simulink model "PubIfDecisionTOS_MDL"  (R2020b)
settings: configuration reference "DspaceConfig" (kept outside this file)
PostLoadFcn:
  | if any(exist('dsrtsu_mdlpostloadfcn', 'file') ~= 0), dsrtsu_mdlpostloadfcn('Execute', bdroot); end
InitFcn:
  | , if any(exist('dsmpb_private', 'file') ~= 0), dsmpb_private('dsmpb_mdlclblib', 'Init', bdroot); end,
undefined symbols (not defined in the file or in its folder): C_TOS_ACCEgoRAxletoFbumplength_m, C_TOS_ACCTargetFront_Flag, C_TOS_AEBJAPedObjDxThre_Val, C_TOS_AEBJAPedObjDyThre_Val, C_TOS_AEBJATargetSize_Val, C_TOS_AEBJAVehObjDxThre_Val, C_TOS_AEBJAVehObjDyThre_Val, C_TOS_AEBJuncPedTargetSize_Val, C_TOS_AEBLatObjDxThre_Val, C_TOS_AEBLatPedDyThre_Val, C_TOS_AEBLatTargetSize_Val, C_TOS_AEBLongTargetInEgoFront_Flag, C_TOS_axAbsGround_Parameter, C_TOS_CameraConfirmedFlag, C_TOS_CNsubjWidth, C_TOS_CurrentLaneCoreMinWidth_Val, C_TOS_CutInProb_Val_Zero, C_TOS_CutOutProb_Val_Zero, C_TOS_D2R_Val, C_TOS_DefaultValueObjectToCenterLine_dy, C_TOS_EgoCarWidth_Val, C_TOS_EgoDxRefPoint_m, C_TOS_EgoRAxletoFbumplength_m, C_TOS_HalfWidthVehicle_Con, C_TOS_HWA_CurrentLaneFlag, C_TOS_HWA_LeftLaneFlag, C_TOS_HWA_MovingDir_Vaild, C_TOS_HWA_MovState_Vaild, C_TOS_HWA_RightLaneFlag, C_TOS_LaneLineCourseErrorFront, C_TOS_LaneLineCourseErrorRear, C_TOS_MotorbikeDefaultWidth_m, C_TOS_NumberOfEffectiveTargets, C_TOS_Obj_Age_Val, C_TOS_Objdx_Constraint_Val, C_TOS_ObjectDefaultWidth_m, C_TOS_ObjInCurrentLane_Val, C_TOS_ObjInCurrentLaneValid, C_TOS_ObjInLeftLaneValid, C_TOS_ObjInRightLaneValid, C_TOS_ObjNotInCurrentLane_Val, C_TOS_ObjNotREElementType, C_TOS_ObjPredictDis_dy_ConstantVal_Zeros, C_TOS_ObjToCenterLine_ConstantVal_Zeros, C_TOS_OFMObjIDInvilad_Val, C_TOS_PIL_LatDisCons_Val_zero, C_TOS_PIL_ObjectCutInFlag_b, C_TOS_PIL_ObjectCutOutFlag_b, C_TOS_PIL_ObjLaneProb_al_Val, C_TOS_PP_ObjFusType_FC_Confirm_b, C_TOS_PP_ObjFusType_FC_FR_Confirm_b, C_TOS_PP_ObjFusType_FR_Confirm_b, C_TOS_RE_80BoolDefault_Val, C_TOS_RE_80Single181Default_Val, C_TOS_RE_80Single255Default_Val, C_TOS_RE_80Uint8Default_Val, C_TOS_RE_D2R, C_TOS_RE_D_180_Val, C_TOS_RE_InvalidObjectID_Val, C_TOS_RE_InvalidTargetChainDir_Val ... (+142)
libraries: simulink x1650, TOS_LIB x361, canfdmsglib x14
(part 1 of 69)
PreSaveFcn:
  | , if any(exist('dsmpb_private', 'file') ~= 0), dsmpb_private('dsmpb_mdlclblib', 'PreSave', bdroot); end,
CloseFcn:
  | , if any(exist('dsmpb_private', 'file') ~= 0), dsmpb_private('dsmpb_mdlclblib', 'Close', bdroot); end,
settings Model: DataDictionary=HWA_DDs.sldd  RTICANMMDATA=struct('GeneralSetupData',struct('modelroot','C:\Users\GW00133806\Desktop\ADAS_Store\Project\V61_Autobox_Noa\LM_TOS','generalsettings',struct('filesettings',struct('destfolder',struct('Name','RTICANMM_FILES','Check',1),'buildfolder',struct('Name','.','Check',1),'AbsDestfolder',struct('Name','C:\Users\GW00133806\Desktop\ADAS_Store\Project\V61_Autobox_Noa\LM_TOS\RTICANMM_FILES'),'AbsBuildfolder',struct('Name','C:\Users\GW00133806\Desktop\ADAS_Store\Project\V61_Autobox_Noa\LM_TOS'))),'options',struct('addpaths',1,'rmpaths',1,'addtrcexclusion',false,'cannavigator',struct('checkmonitoring',0),'show_usrtrc',0,'use_usrtrc',0),'advanced',struct('options',ones(1,100)),'MPSetup',{{}},'RTI',struct('Type','DSRT','Ver','4.2','Date','02-Nov-2019'),'modelname','PubIfDecisionTOS_MDL','block','PubIfDecisionTOS_MDL'))  DSRTSU_INTERNAL_RTIFPGA=150  Creator=GW00180895  LastModifiedBy=GW00133806
settings ConfigSetRef: SourceName=DspaceConfig

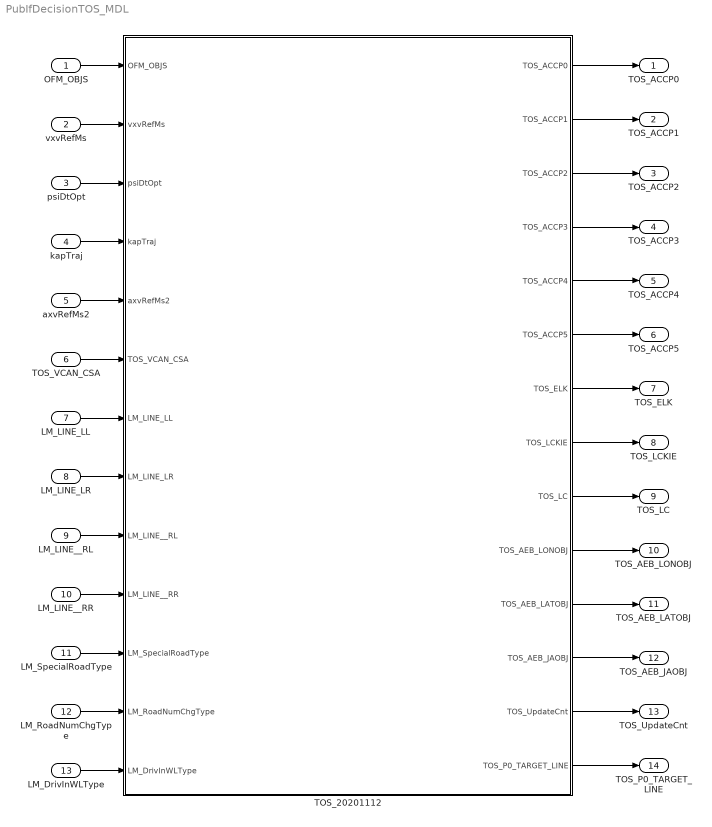
== system PubIfDecisionTOS_MDL ==
  OFM_OBJS : Inport  OutDataTypeStr=Bus: OFM_OBJ_BUS  PortDimensions=1  BusOutputAsStruct=on
  vxvRefMs : Inport  Port=2  OutDataTypeStr=single  PortDimensions=1  BusOutputAsStruct=on
  psiDtOpt : Inport  Port=3  OutDataTypeStr=single  PortDimensions=1  BusOutputAsStruct=on
  kapTraj : Inport  Port=4  OutDataTypeStr=single  PortDimensions=1  BusOutputAsStruct=on
  axvRefMs2 : Inport  Port=5  OutDataTypeStr=single  PortDimensions=1  BusOutputAsStruct=on
  TOS_VCAN_CSA : Inport  Port=6  OutDataTypeStr=Bus: TOS_VCAN_CSA_BUS  BusOutputAsStruct=on
  LM_LINE_LL : Inport  Port=7  OutDataTypeStr=Bus: LM_LINE_BUS  PortDimensions=1  BusOutputAsStruct=on
  LM_LINE_LR : Inport  Port=8  OutDataTypeStr=Bus: LM_LINE_BUS  PortDimensions=1  BusOutputAsStruct=on
  LM_LINE__RL : Inport  Port=9  OutDataTypeStr=Bus: LM_LINE_BUS  PortDimensions=1  BusOutputAsStruct=on
  LM_LINE__RR : Inport  Port=10  OutDataTypeStr=Bus: LM_LINE_BUS  PortDimensions=1  BusOutputAsStruct=on
  LM_SpecialRoadType : Inport  Port=11  OutDataTypeStr=uint8  PortDimensions=1  BusOutputAsStruct=on
  LM_RoadNumChgType : Inport  Port=12  OutDataTypeStr=uint8  PortDimensions=1  BusOutputAsStruct=on
  LM_DrivInWLType : Inport  Port=13  OutDataTypeStr=uint8  PortDimensions=1  BusOutputAsStruct=on
  TOS_20201112 : Subsystem
  TOS_ACCP0 : Outport  OutDataTypeStr=Bus: TOS_ACCP0_BUS  PortDimensions=1  BusOutputAsStruct=on
  TOS_ACCP1 : Outport  Port=2  OutDataTypeStr=Bus: TOS_ACCP1_BUS  PortDimensions=1  BusOutputAsStruct=on
  TOS_ACCP2 : Outport  Port=3  OutDataTypeStr=Bus: TOS_ACCP2_BUS  PortDimensions=1  BusOutputAsStruct=on
  TOS_ACCP3 : Outport  Port=4  OutDataTypeStr=Bus: TOS_ACCP3_BUS  PortDimensions=1  BusOutputAsStruct=on
  TOS_ACCP4 : Outport  Port=5  OutDataTypeStr=Bus: TOS_ACCP4_BUS  PortDimensions=1  BusOutputAsStruct=on
  TOS_ACCP5 : Outport  Port=6  OutDataTypeStr=Bus: TOS_ACCP5_BUS  PortDimensions=1  BusOutputAsStruct=on
  TOS_ELK : Outport  Port=7  OutDataTypeStr=Bus: TOS_ELK_BUS  PortDimensions=1  BusOutputAsStruct=on
  TOS_LCKIE : Outport  Port=8  OutDataTypeStr=Bus: TOS_LCKIE_BUS  PortDimensions=1  BusOutputAsStruct=on
  TOS_LC : Outport  Port=9  OutDataTypeStr=Bus: TOS_LC_BUS  PortDimensions=1  BusOutputAsStruct=on
  TOS_AEB_LONOBJ : Outport  Port=10  OutDataTypeStr=Bus: TOS_AEB_LONOBJ_BUS  PortDimensions=1  BusOutputAsStruct=on
  TOS_AEB_LATOBJ : Outport  Port=11  OutDataTypeStr=Bus: TOS_AEB_LATOBJ_BUS  PortDimensions=10  BusOutputAsStruct=on
  TOS_AEB_JAOBJ : Outport  Port=12  OutDataTypeStr=Bus: TOS_AEB_JAOBJ_BUS  PortDimensions=32  BusOutputAsStruct=on
  TOS_UpdateCnt : Outport  Port=13  OutDataTypeStr=uint32  PortDimensions=1  BusOutputAsStruct=on
  TOS_P0_TARGET_LINE : Outport  Port=14  OutDataTypeStr=Bus: TOS_P0_TARGET_LINE_BUS  PortDimensions=1  BusOutputAsStruct=on
  wires:
  OFM_OBJS/1 -> TOS_20201112/1(OFM_OBJS)
  vxvRefMs/1 -> TOS_20201112/2(vxvRefMs)
  psiDtOpt/1 -> TOS_20201112/3(psiDtOpt)
  kapTraj/1 -> TOS_20201112/4(kapTraj)
  axvRefMs2/1 -> TOS_20201112/5(axvRefMs2)
  TOS_VCAN_CSA/1 -> TOS_20201112/6(TOS_VCAN_CSA)
  LM_LINE_LL/1 -> TOS_20201112/7(LM_LINE_LL)
  LM_LINE_LR/1 -> TOS_20201112/8(LM_LINE_LR)
  LM_LINE__RL/1 -> TOS_20201112/9(LM_LINE__RL)
  LM_LINE__RR/1 -> TOS_20201112/10(LM_LINE__RR)
  LM_SpecialRoadType/1 -> TOS_20201112/11(LM_SpecialRoadType)
  LM_RoadNumChgType/1 -> TOS_20201112/12(LM_RoadNumChgType)
  LM_DrivInWLType/1 -> TOS_20201112/13(LM_DrivInWLType)
  TOS_20201112/2(TOS_ACCP1) -> TOS_ACCP1/1
  TOS_20201112/1(TOS_ACCP0) -> TOS_ACCP0/1
  TOS_20201112/3(TOS_ACCP2) -> TOS_ACCP2/1
  TOS_20201112/4(TOS_ACCP3) -> TOS_ACCP3/1
  TOS_20201112/5(TOS_ACCP4) -> TOS_ACCP4/1
  TOS_20201112/6(TOS_ACCP5) -> TOS_ACCP5/1
  TOS_20201112/7(TOS_ELK) -> TOS_ELK/1
  TOS_20201112/8(TOS_LCKIE) -> TOS_LCKIE/1
  TOS_20201112/9(TOS_LC) -> TOS_LC/1
  TOS_20201112/10(TOS_AEB_LONOBJ) -> TOS_AEB_LONOBJ/1
  TOS_20201112/11(TOS_AEB_LATOBJ) -> TOS_AEB_LATOBJ/1
  TOS_20201112/12(TOS_AEB_JAOBJ) -> TOS_AEB_JAOBJ/1
  TOS_20201112/13(TOS_UpdateCnt) -> TOS_UpdateCnt/1
  TOS_20201112/14(TOS_P0_TARGET_LINE) -> TOS_P0_TARGET_LINE/1

== system PubIfDecisionTOS_MDL/TOS_20201112 ==
  OFM_OBJS : Inport  OutDataTypeStr=Bus: OFM_OBJ_BUS  PortDimensions=1  BusOutputAsStruct=on
  vxvRefMs : Inport  Port=2  OutDataTypeStr=single  PortDimensions=1  BusOutputAsStruct=on
  psiDtOpt : Inport  Port=3  OutDataTypeStr=single  PortDimensions=1  BusOutputAsStruct=on
  kapTraj : Inport  Port=4  OutDataTypeStr=single  PortDimensions=1  BusOutputAsStruct=on
  axvRefMs2 : Inport  Port=5  OutDataTypeStr=single  PortDimensions=1  BusOutputAsStruct=on
  TOS_VCAN_CSA : Inport  Port=6  OutDataTypeStr=Bus: TOS_VCAN_CSA_BUS  BusOutputAsStruct=on
  LM_LINE_LL : Inport  Port=7  OutDataTypeStr=Bus: LM_LINE_BUS  PortDimensions=1  BusOutputAsStruct=on
  LM_LINE_LR : Inport  Port=8  OutDataTypeStr=Bus: LM_LINE_BUS  PortDimensions=1  BusOutputAsStruct=on
  LM_LINE__RL : Inport  Port=9  OutDataTypeStr=Bus: LM_LINE_BUS  PortDimensions=1  BusOutputAsStruct=on
  LM_LINE__RR : Inport  Port=10  OutDataTypeStr=Bus: LM_LINE_BUS  PortDimensions=1  BusOutputAsStruct=on
  LM_SpecialRoadType : Inport  Port=11  OutDataTypeStr=uint8  PortDimensions=1  BusOutputAsStruct=on
  LM_RoadNumChgType : Inport  Port=12  OutDataTypeStr=uint8  PortDimensions=1  BusOutputAsStruct=on
  LM_DrivInWLType : Inport  Port=13  OutDataTypeStr=uint8  PortDimensions=1  BusOutputAsStruct=on
  Constant : Constant  Value=2011100315  OutDataTypeStr=uint32
  Model Info : simulink/Model-Wide Utilities/Model Info  Frame=on  DisplayStringWithTags=|  HorizontalTextAlignment=Left  LeftAlignmentValue=0.02
      | 2020/11/3
      | 1】 优化PIL模型,将目标在三个车道概率值归一化为1
      | 2】目标所在车道PIL概率计算（独立事件求和）
      | 3】自车所在车道概率值计算、均值滤波
      | 4】目标所在车道判断TLJ模块优化
      | 5】LM输入车道线信息变更
      | 6】cut in 目标宽度约束 2020/11/04
      | 7】TLJ添加cut in/cut out 目标判断逻辑 2020/11/04
      | 8】cut out / in 只对运动目标预测、根据VY速度约束vyc值 2020/11/04
      | 
      | 2020/11/09
      | 1】ACC（P0、P1）静止目标dx<90m,运动目标dx<120m
      | 2】ACC（P0、P1）dy约束Car 的1.9m<dy<1.8m 内，静止目标dy约束在1.5m<dy<1.45m 内（间隔20m）dy约束行人的1.4m<dy<1.2m 内，
      | 
      | 2020/11/10
      | 1】 cut in/out 集成最新版（只对运动目标判断切入/出）
      | 
      | 2020/11/12
      | 1】ACC（P0、P1）静止目标dx<90m,运动目标dx<120m
      | 2】ACC（P0、P1）dy约束（静止、运动到静止、未知）Car、truck 的 1.6m→1.5m 内，
      |     ACC（P0、P1）dy约束（运动、低速运动）Car、truck 的 1.8m→1.7m 内，
      |     行人、自行车、摩托车、未知类型 目标dy约束在1.4m→1.2m 内
      |     其他目标：1.4m→1.2m
      | 3】优化HWA目标选择策略，左右车道、本车道后方目标
  Model Info1 : simulink/Model-Wide Utilities/Model Info  Frame=on  DisplayStringWithTags=|  HorizontalTextAlignment=Left  LeftAlignmentValue=0.02
      | 2020/11/10
      | 1】 过滤目标：选中目标后，此补丁用于去掉突然出现的纵向距离更近的单雷达静止目标
      |     TOS/ACC/TOS_ACCCurrentLane/ACC_Object_PreJudge
      |     TOS/AEB/TOS_AEBLong/AEBLong_Target_PreJudge
      | 
      | 2]延时3帧模块
      | TOS/ACC/TOS_ACCCurrentLane/ACC_CurrentLane_Target
      | //TOS_ACC_FusionType//TOS_ACC_TargetMovingDir//TOS_ACC_ObjType//TOS_ACC_ObstacleConfirm
      | TOS/AEB/TOS_AEBLong/AEBLong_Confirm 
      | //TOS_AEBLong_ObstacleProb//TOS_AEBLong_ObjFusType//TOS_AEBLong_TargetMovingDir
      | 
      | 3]针对连续3帧选中的运动（或运动到静止）目标，改变其运动状态一直为运动（或运动到静止）
      | TOS/ACC/TOS_ACCCurrentLane/ACC_CurrentLane_Target
      | //TOS_ACC_FusionTypeTOS_ACC_ObjType
      | TOS/AEB/TOS_AEBLong/AEBLong_Confirm 
      | //TOS_AEBLong_ObjFusType
      | 
      | 4]已选中目标，前两个周期为运动，以后为运动，前两个周期为Stopped，以后为Stopped
      | TOS/ACC/TOS_ACCCurrentLane/ACC_CurrentLane_Target
      | //TOS_ACC_TargetMovingDir
      | TOS/AEB/TOS_AEBLong/AEBLong_Confirm 
      | //TOS_ACC_TargetMovingDir
  TOS_2012080320 : Subsystem
  Terminator : Terminator
  TOS_ACCP0 : Outport  OutDataTypeStr=Bus: TOS_ACCP0_BUS  PortDimensions=1  BusOutputAsStruct=on
  TOS_ACCP1 : Outport  Port=2  OutDataTypeStr=Bus: TOS_ACCP1_BUS  PortDimensions=1  BusOutputAsStruct=on
  TOS_ACCP2 : Outport  Port=3  OutDataTypeStr=Bus: TOS_ACCP2_BUS  PortDimensions=1  BusOutputAsStruct=on
  TOS_ACCP3 : Outport  Port=4  OutDataTypeStr=Bus: TOS_ACCP3_BUS  PortDimensions=1  BusOutputAsStruct=on
  TOS_ACCP4 : Outport  Port=5  OutDataTypeStr=Bus: TOS_ACCP4_BUS  PortDimensions=1  BusOutputAsStruct=on
  TOS_ACCP5 : Outport  Port=6  OutDataTypeStr=Bus: TOS_ACCP5_BUS  PortDimensions=1  BusOutputAsStruct=on
  TOS_ELK : Outport  Port=7  OutDataTypeStr=Bus: TOS_ELK_BUS  PortDimensions=1  BusOutputAsStruct=on
  TOS_LCKIE : Outport  Port=8  OutDataTypeStr=Bus: TOS_LCKIE_BUS  PortDimensions=1  BusOutputAsStruct=on
  TOS_LC : Outport  Port=9  OutDataTypeStr=Bus: TOS_LC_BUS  PortDimensions=1  BusOutputAsStruct=on
  TOS_AEB_LONOBJ : Outport  Port=10  OutDataTypeStr=Bus: TOS_AEB_LONOBJ_BUS  PortDimensions=1  BusOutputAsStruct=on
  TOS_AEB_LATOBJ : Outport  Port=11  OutDataTypeStr=Bus: TOS_AEB_LATOBJ_BUS  PortDimensions=10  BusOutputAsStruct=on
  TOS_AEB_JAOBJ : Outport  Port=12  OutDataTypeStr=Bus: TOS_AEB_JAOBJ_BUS  PortDimensions=32  BusOutputAsStruct=on
  TOS_UpdateCnt : Outport  Port=13  OutDataTypeStr=uint32  PortDimensions=1  BusOutputAsStruct=on
  TOS_P0_TARGET_LINE : Outport  Port=14  OutDataTypeStr=Bus: TOS_P0_TARGET_LINE_BUS  PortDimensions=1  BusOutputAsStruct=on
  wires:
  TOS_2012080320/14(TOS_UpdateCnt) -> TOS_UpdateCnt/1
  TOS_2012080320/8(TOS_ACCP4) -> TOS_ACCP4/1
  TOS_2012080320/7(TOS_ACCP3) -> TOS_ACCP3/1
  TOS_2012080320/6(TOS_ACCP2) -> TOS_ACCP2/1
  TOS_2012080320/11(TOS_LCKIE) -> TOS_LCKIE/1
  TOS_2012080320/12(TOS_ELK) -> TOS_ELK/1
  TOS_2012080320/9(TOS_ACCP5) -> TOS_ACCP5/1
  LM_LINE_LL/1 -> TOS_2012080320/7(LM_LINE_LL)
  kapTraj/1 -> TOS_2012080320/4(kapTraj)
  psiDtOpt/1 -> TOS_2012080320/3(psiDtOpt)
  vxvRefMs/1 -> TOS_2012080320/2(vxvRefMs)
  LM_LINE_LR/1 -> TOS_2012080320/8(LM_LINE_LR)
  TOS_2012080320/3(TOS_AEB_LATOBJ) -> TOS_AEB_LATOBJ/1
  TOS_2012080320/2(TOS_AEB_JAOBJ) -> TOS_AEB_JAOBJ/1
  LM_DrivInWLType/1 -> TOS_2012080320/13(LM_DrivInWLType)
  TOS_2012080320/1(TOS_AEBLONOBJ) -> TOS_AEB_LONOBJ/1
  LM_RoadNumChgType/1 -> TOS_2012080320/12(LM_RoadNumChgType)
  LM_LINE__RR/1 -> TOS_2012080320/10(LM_LINE_RR)
  TOS_VCAN_CSA/1 -> TOS_2012080320/6(TOS_VCAN_CSA)
  OFM_OBJS/1 -> TOS_2012080320/1(OFM_OBJS)  "OFM_OBJS"
  TOS_2012080320/10(TOS_LC) -> TOS_LC/1
  LM_LINE__RL/1 -> TOS_2012080320/9(LM_LINE_RL)
  TOS_2012080320/4(TOS_ACCP0) -> TOS_ACCP0/1
  TOS_2012080320/5(TOS_ACCP1) -> TOS_ACCP1/1
  axvRefMs2/1 -> TOS_2012080320/5(axvRefMs2)
  TOS_2012080320/13(TOS_P0_TARGET_LINE) -> TOS_P0_TARGET_LINE/1
  LM_SpecialRoadType/1 -> TOS_2012080320/11(LM_SpecialRoadType)
  Constant/1 -> Terminator/1  "TOS_SW_VERSION"

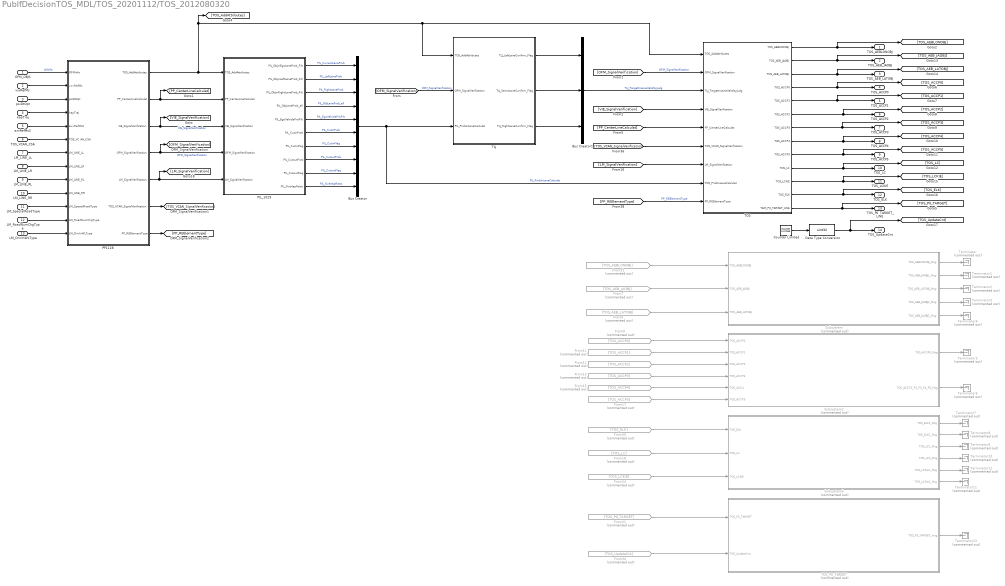
== system PubIfDecisionTOS_MDL/TOS_20201112/TOS_2012080320 ==
  OFM_OBJS : Inport  PortDimensions=1  BusOutputAsStruct=on
  vxvRefMs : Inport  Port=2
  psiDtOpt : Inport  Port=3  Interpolate=off
  kapTraj : Inport  Port=4
  axvRefMs2 : Inport  Port=5  OutDataTypeStr=single
  TOS_VCAN_CSA : Inport  Port=6  BusOutputAsStruct=on
  LM_LINE_LL : Inport  Port=7  BusOutputAsStruct=on
  LM_LINE_LR : Inport  Port=8  BusOutputAsStruct=on
  LM_LINE_RL : Inport  Port=9  BusOutputAsStruct=on
  LM_LINE_RR : Inport  Port=10  BusOutputAsStruct=on
  LM_SpecialRoadType : Inport  Port=11  OutDataTypeStr=uint8  PortDimensions=1  BusOutputAsStruct=on
  LM_RoadNumChgType : Inport  Port=12  OutDataTypeStr=uint8  PortDimensions=1  BusOutputAsStruct=on
  LM_DrivInWLType : Inport  Port=13  OutDataTypeStr=uint8  PortDimensions=1  BusOutputAsStruct=on
  Bus Creator : BusCreator  Inputs=10  OutDataTypeStr=Bus: PIL_ProbInLaneCalculat_BUS  NonVirtualBus=on
      settings: InheritFromInputs=off
  Bus Creator1 : BusCreator  Inputs=3
  Counter Limited : simulink/Sources/Counter Limited  uplimit=255  tsamp=-1
  Data Type Conversion : DataTypeConversion  OutDataTypeStr=uint32
  From11 : From  Commented=on  GotoTag=TOS_ACCP1
  From12 : From  Commented=on  GotoTag=TOS_ACCP2
  From13 : From  Commented=on  GotoTag=TOS_ACCP3
  From15 : From  Commented=on  GotoTag=TOS_ACCP4
  From17 : From  Commented=on  GotoTag=TOS_ACCP5
  From18 : From  Commented=on  GotoTag=TOS_LC
  From21 : From  Commented=on  GotoTag=TOS_P0_TARGET
  From24 : From  Commented=on  GotoTag=TOS_LCKIE
  From30 : From  Commented=on  GotoTag=TOS_ELK
  From31 : From  Commented=on  GotoTag=TOS_AEBLONOBJ
  From34 : From  Commented=on  GotoTag=TOS_UpdateCnt
  From7 : From  Commented=on  GotoTag=TOS_AEB_JAOBJ
  From8 : From  Commented=on  GotoTag=TOS_AEB_LATOBJ
  From9 : From  Commented=on  GotoTag=TOS_ACCP0
  PIL_1029 : Subsystem
  PP1128 : Subsystem
  Subsystem : Subsystem  Commented=on
  Subsystem2 : Subsystem  Commented=on
  Subsystem3 : Subsystem  Commented=on
  TLJ : Subsystem
  TOS : Subsystem
  TOS_P0_TARGET : Subsystem  Commented=on
  Terminator{,1..13} (14 alike) : Terminator  Commented=on
  TOS_AEBLONOBJ : Outport  PortDimensions=1  BusOutputAsStruct=on
  TOS_AEB_JAOBJ : Outport  Port=2  BusOutputAsStruct=on
  TOS_AEB_LATOBJ : Outport  Port=3  BusOutputAsStruct=on
  TOS_ACCP0 : Outport  Port=4  PortDimensions=1  BusOutputAsStruct=on
  TOS_ACCP1 : Outport  Port=5  PortDimensions=1  BusOutputAsStruct=on
  TOS_ACCP2 : Outport  Port=6  PortDimensions=1  BusOutputAsStruct=on
  TOS_ACCP3 : Outport  Port=7  PortDimensions=1  BusOutputAsStruct=on
  TOS_ACCP4 : Outport  Port=8  PortDimensions=1  BusOutputAsStruct=on
  TOS_ACCP5 : Outport  Port=9  PortDimensions=1  BusOutputAsStruct=on
  TOS_LC : Outport  Port=10  PortDimensions=1  BusOutputAsStruct=on
  TOS_LCKIE : Outport  Port=11  PortDimensions=1  BusOutputAsStruct=on
  TOS_ELK : Outport  Port=12  PortDimensions=1  BusOutputAsStruct=on
  TOS_P0_TARGET_LINE : Outport  Port=13  PortDimensions=1  BusOutputAsStruct=on
  TOS_UpdateCnt : Outport  Port=14  OutDataTypeStr=uint32  PortDimensions=1  BusOutputAsStruct=on
  wires:
  psiDtOpt/1 -> PP1128/3(psiDtOpt)
  vxvRefMs/1 -> PP1128/2(vxvRefMs)
  kapTraj/1 -> PP1128/4(kapTraj)
  TOS_VCAN_CSA/1 -> PP1128/6(TOS_VC AN_CSA)
  axvRefMs2/1 -> PP1128/5(axvRefMs2)
  TOS/2(TOS_AEB_JAOBJ) -> [TOS_AEB_JAOBJ], TOS_AEB_JAOBJ/1
  TOS/3(TOS_AEB_LATOBJ) -> [TOS_AEB_LATOBJ], TOS_AEB_LATOBJ/1
  TOS/4(TOS_ACCP0) -> [TOS_ACCP0], TOS_ACCP0/1
  TOS/5(TOS_ACCP1) -> [TOS_ACCP1], TOS_ACCP1/1
  TOS/6(TOS_ACCP2) -> [TOS_ACCP2], TOS_ACCP2/1
  TOS/7(TOS_ACCP3) -> [TOS_ACCP3], TOS_ACCP3/1
  TOS/8(TOS_ACCP4) -> [TOS_ACCP4], TOS_ACCP4/1
  TOS/9(TOS_ACCP5) -> [TOS_ACCP5], TOS_ACCP5/1
  TOS/10(TOS_LC) -> [TOS_LC], TOS_LC/1
  TOS/11(TOS_LCKIE) -> [TOS_LCKIE], TOS_LCKIE/1
  TOS/12(TOS_ELK) -> [TOS_ELK], TOS_ELK/1
  TOS/13(TEM_P0_TARGET_LINE) -> [TOS_P0_TARGET], TOS_P0_TARGET_LINE/1
  Counter Limited/1 -> Data Type Conversion/1
  LM_LINE_LL/1 -> PP1128/7(LM_LINE_LL)
  LM_LINE_LR/1 -> PP1128/8(LM_LINE_LR)
  LM_LINE_RL/1 -> PP1128/9(LM_LINE_RL)
  LM_LINE_RR/1 -> PP1128/10(LM_LINE_RR)
  LM_SpecialRoadType/1 -> PP1128/11(LM_SpecialRoadType)
  LM_RoadNumChgType/1 -> PP1128/12(LM_RoadNumChgType)
  LM_DrivInWLType/1 -> PP1128/13(LM_DrivInWLType)
  OFM_OBJS/1 -> PP1128/1(OFMInfo)  "LMInfo"
  TOS/1(TOS_AEBLONOBJ) -> [TOS_AEBLONOBJ], TOS_AEBLONOBJ/1
  PIL_1029/8(PIL_CutoutProb) -> Bus Creator/8  "PIL_CutoutProb"
  TLJ/3(TLJ_RightLaneConfirm_Flag) -> Bus Creator1/3
  PIL_1029/7(PIL_CutinFlag) -> Bus Creator/7  "PIL_CutinFlag"
  Bus Creator1/1 -> TOS/3(TLJ_TargetInLaneValidityJudg)  "TLJ_TargetInLaneValidityJudg"
  [OFM_SignalVerification] -> TOS/2(OFM_SignalVerification)  "OFM_SignalVerification"
  Bus Creator/1 -> TLJ/3(PIL_ProbInLaneCalculat), TOS/8(TOS_ProbInLaneCalculat)  "PIL_ProbInLaneCalculat"
  [PP_CenterLineCalculat] -> TOS/5(PP_CenterLineCalculat)
  PP1128/2(PP_CenterLineCalculat) -> [PP_CenterLineCalculat], PIL_1029/2(PP_CenterLineCalculat)
  PIL_1029/2(PIL_ObjinLeftLaneProb_Filt) -> Bus Creator/2  "PIL_LeftLaneProb"
  PIL_1029/9(PIL_CutoutFlag) -> Bus Creator/9  "PIL_CutoutFlag"
  PIL_1029/3(PIL_ObjinRightLaneProb_Filt) -> Bus Creator/3  "PIL_RightLaneProb"
  [VIE_SignalVerification] -> TOS/4(VIE_SignalVerification)
  PP1128/3(VIE_SignalVerification) -> [VIE_SignalVerification], PIL_1029/3(VIE_SignalVerification)  "VIE_SignalVerification"
  PP1128/4(OFM_SignalVerification) -> PIL_1029/4("OFM_SignalVerification "), [OFM_SignalVerification]  "OFM_SignalVerification"
  PIL_1029/1(PIL_ObjinEgoLaneProb_Filt) -> Bus Creator/1  "PIL_CurrentLaneProb"
  TLJ/1(TLJ_LeftLaneConfirm_Flag) -> Bus Creator1/1
  PIL_1029/6(PIL_CutinProb) -> Bus Creator/6  "PIL_CutinProb"
  [OFM_SignalVerification] -> TLJ/2(OFM_SignalVerification)  "OFM_SignalVerification"
  PP1128/1(TOS_AddAttributes) -> [TOS_AddAttributes], TLJ/1(TOS_AddAttributes), TOS/1(TOS_AddAttributes), PIL_1029/1(TOS_AddAttributes)
  PP1128/5(LM_SignalVerification) -> [LM_SignalVerification], PIL_1029/5(LM_SignalVerification)
  From31/1 -> Subsystem/1(TOS_AEBLONOBJ)
  From7/1 -> Subsystem/2(TOS_AEB_JAOBJ)
  From8/1 -> Subsystem/3(TOS_AEB_LATOBJ)
  From11/1 -> Subsystem2/2(TOS_ACCP1)
  From9/1 -> Subsystem2/1(TOS_ACCP0)
  From12/1 -> Subsystem2/3(TOS_ACCP2)
  From13/1 -> Subsystem2/4(TOS_ACCP3)
  From15/1 -> Subsystem2/5(TOS_ACC4)
  From17/1 -> Subsystem2/6(TOS_ACCP5)
  From30/1 -> Subsystem3/1(TOS_ELK)
  From18/1 -> Subsystem3/2(TOS_LC)
  From24/1 -> Subsystem3/3(TOS_LCKIE)
  Subsystem/1(TOS_AEBLONOBJ_Msg) -> Terminator/1
  Subsystem/2(TOS_AEB_JAOBJ1_Msg) -> Terminator1/1
  Subsystem/3(TOS_AEB_LATOBJ_Msg) -> Terminator2/1
  Subsystem/4(TOS_AEB_JAOBJ2_Msg) -> Terminator3/1
  Subsystem/5(TOS_AEB_JAOBJ3_Msg) -> Terminator4/1
  Subsystem2/1(TOS_ACCP0_Msg) -> Terminator5/1
  Subsystem2/2(TOS_ACCP1_P2_P3_P4_P5_Msg) -> Terminator6/1
  Subsystem3/1(TOS_ELK1_Msg) -> Terminator7/1
  Subsystem3/2(TOS_ELK2_Msg) -> Terminator8/1
  Subsystem3/3(TOS_LC1_Msg) -> Terminator9/1
  Subsystem3/4(TOS_LC2_Msg) -> Terminator10/1
  Subsystem3/5(TOS_LCKie1_Msg) -> Terminator12/1
  Subsystem3/6(TOS_LCKie2_Msg) -> Terminator11/1
  PP1128/6(TOS_VCAN_SignalVerification) -> [TOS_VCAN_SignalVerification]
  [TOS_VCAN_SignalVerification] -> TOS/6(TOS_VCAN_SignalVerification)
  From21/1 -> TOS_P0_TARGET/1(TOS_P0_TARGET)
  TOS_P0_TARGET/1(TOS_P0_TARGET_msg) -> Terminator13/1
  From34/1 -> TOS_P0_TARGET/2(TOS_UpdateCnt)
  PIL_1029/10(PIL_OverlapRatio) -> Bus Creator/10  "PIL_OverlapRatio"
  Data Type Conversion/1 -> [TOS_UpdateCnt], TOS_UpdateCnt/1
  PIL_1029/5(PIL_EgoVehicleProFilt) -> Bus Creator/5  "PIL_EgoVehicleProFilt"
  TLJ/2(TLJ_SameLaneConfirm_Flag) -> Bus Creator1/2
  PIL_1029/4("PIL_ObjLaneProb_all ") -> Bus Creator/4  "PIL_ObjLaneProb_all"
  [LM_SignalVerification] -> TOS/7(LM_SignalVerification)
  PP1128/7(PP_REElementType) -> [PP_REElementType]
  [PP_REElementType] -> TOS/9(PP_REElementType)  "PP_REElementType"

== system PubIfDecisionTOS_MDL/TOS_20201112/TOS_2012080320/PIL_1029 ==
  TOS_AddAttributes : Inport
  PP_CenterLineCalculat : Inport  Port=2
  VIE_SignalVerification : Inport  Port=3
  "OFM_SignalVerification " : Inport  Port=4
  LM_SignalVerification : Inport  Port=5
  BoundaryCalculat : Subsystem
  Bus Creator : BusCreator  Inputs=2
  Bus Creator1 : BusCreator  Inputs=5
  Bus Selector2 : BusSelector  OutputSignals=TOS_PP_AddAttributes_bus.PP_ObjectToCenterLine_dy,OFM_SignalVerification.TOS_OFMObjValid_Flag,OFM_SignalVerification.Object_ID,OFM_SignalVerification.Object_Age
  Bus Selector3 : BusSelector  OutputSignals=OFM_SignalVerification,TOS_PP_AddAttributes_bus,PP_CenterLineCalculat.signal4
  Bus Selector5 : BusSelector  OutputSignals=PIL_Lane_BoundaryCalculat,PIL_ObjectToCenterLine_dyc
  Bus Selector6 : BusSelector  OutputSignals=OFM_SignalVerification.TOS_OFMObjValid_Flag,OFM_SignalVerification.Object_Width,TOS_PP_AddAttributes_bus.PP_CamareConfirmSignalProcessing,OFM_SignalVerification.Object_MovingState,OFM_SignalVerification.Object_Type,TOS_PP_AddAttributes_bus.PP_EgoVehCenterLine_dy,TOS_PP_AddAttributes_bus.PP_ObjectToCenterLine_dy
  Bus Selector7 : BusSelector  OutputSignals=PP_CenterLineCalculat.PP_EgoLane_CenterLine,OFM_SignalVerification,TOS_PP_AddAttributes_bus,LM_SignalVerification
  Bus Selector8 : BusSelector  OutputSignals=OFM_SignalVerification,TOS_PP_AddAttributes_bus,PP_CenterLineCalculat.PP_EgoLane_CenterLine,PP_CenterLineCalculat.PP_LeftLane_CenterLine,PP_CenterLineCalculat.PP_RightLane_CenterLine,PP_CenterLineCalculat.signal4
  ObjCutInOut_Prob : Subsystem
  OverlapRatio_Calculate : Subsystem
  PIL_ObjectToCenterLine_dy_Filt : Subsystem
  ProbCalculat : Subsystem
  PIL_ObjinEgoLaneProb_Filt : Outport  OutDataTypeStr=single
  PIL_ObjinLeftLaneProb_Filt : Outport  Port=2  OutDataTypeStr=single
  PIL_ObjinRightLaneProb_Filt : Outport  Port=3  OutDataTypeStr=single
  "PIL_ObjLaneProb_all " : Outport  Port=4
  PIL_EgoVehicleProFilt : Outport  Port=5
  PIL_CutinProb : Outport  Port=6  OutDataTypeStr=single
  PIL_CutinFlag : Outport  Port=7  OutDataTypeStr=boolean
  PIL_CutoutProb : Outport  Port=8  OutDataTypeStr=single
  PIL_CutoutFlag : Outport  Port=9  OutDataTypeStr=boolean
  PIL_OverlapRatio : Outport  Port=10  OutDataTypeStr=single
  wires:
  Bus Creator1/1 -> [PIL_InPutSig], Bus Selector8/1, Bus Selector2/1, Bus Selector6/1
  Bus Selector6/3 -> OverlapRatio_Calculate/3(ObjectTypeCameraConfirmed)  "<PP_CamareConfirmSignalProcessing>"
  OverlapRatio_Calculate/1(PIL_OverlapRatio) -> PIL_OverlapRatio/1  "TOS_PIL_OverlapRatio"
  Bus Selector6/1 -> OverlapRatio_Calculate/1(TOS_OFMObjValid_Flag)  "<TOS_OFMObjValid_Flag>"
  Bus Selector6/6 -> OverlapRatio_Calculate/6(dyEgo2Center)  "<PP_EgoVehCenterLine_dy>"
  Bus Selector6/2 -> OverlapRatio_Calculate/2(ObjectWidth)  "<Object_Width>"
  Bus Selector6/4 -> OverlapRatio_Calculate/4(object_MovingState)  "<Object_MovingState>"
  Bus Selector6/7 -> OverlapRatio_Calculate/7(dyObject2Center)  "<PP_ObjectToCenterLine_dy>"
  Bus Selector5/2 -> ProbCalculat/6(PIL_ObjectToCenterLine_dyc)  "<PIL_ObjectToCenterLine_dyc>"
  Bus Selector5/1 -> ProbCalculat/5(PIL_Lane_BoundaryCalculat)  "<PIL_Lane_BoundaryCalculat>"
  BoundaryCalculat/2(PIL_ObjectToCenterLine_dyc) -> Bus Creator/2
  Bus Selector2/2 -> PIL_ObjectToCenterLine_dy_Filt/2(TOS_OFMObjValid_Flag)  "<TOS_OFMObjValid_Flag>"
  Bus Selector2/4 -> PIL_ObjectToCenterLine_dy_Filt/4(Object_Age)  "<Object_Age>"
  LM_SignalVerification/1 -> Bus Creator1/5
  Bus Selector3/3 -> ObjCutInOut_Prob/4(LaneWidth)  "<signal4>"
  Bus Selector7/1 -> ProbCalculat/1(CurrentLane_LeftRightLine)  "<PP_EgoLane_CenterLine>"
  Bus Selector8/6 -> BoundaryCalculat/6(PP_CenterLineCalculat)  "<signal4>"
  Bus Selector7/3 -> ProbCalculat/3(TOS_AddAttributes)  "<TOS_PP_AddAttributes_bus>"
  Bus Selector3/2 -> ObjCutInOut_Prob/3(TOS_AddAttributes)  "<TOS_PP_AddAttributes_bus>"
  Bus Selector3/1 -> ObjCutInOut_Prob/2(OFM_SignalVerification)  "<OFM_SignalVerification>"
  [PIL_InPutSig] -> Bus Selector3/1
  ObjCutInOut_Prob/4(PIL_ObjectCutOutFlag) -> PIL_CutoutFlag/1
  ObjCutInOut_Prob/3(PIL_ObjectCutOutPro) -> PIL_CutoutProb/1
  ObjCutInOut_Prob/2(PIL_ObjectCutIn_Flag) -> PIL_CutinFlag/1
  ObjCutInOut_Prob/1(PIL_ObjectCutInPro_Filt) -> PIL_CutinProb/1
  PIL_ObjectToCenterLine_dy_Filt/1(PIL_ObjectToCenterLine_dy_Filt) -> ObjCutInOut_Prob/1(PIL_ObjectToCenterLine_dy_Filt)  "PIL_ObjectToCenterLine_dy_Filt"
  Bus Selector7/2 -> ProbCalculat/2(OFM_SignalVerification)  "<OFM_SignalVerification>"
  [PIL_InPutSig] -> Bus Selector7/1
  BoundaryCalculat/1(PIL_Lane_BoundaryCalculat) -> Bus Creator/1
  Bus Creator/1 -> [BoundaryCalculat], Bus Selector5/1
  ProbCalculat/3(PIL_ObjinRightLaneProb_Filt) -> PIL_ObjinRightLaneProb_Filt/1
  ProbCalculat/2(PIL_ObjinLeftLaneProb_Filt) -> PIL_ObjinLeftLaneProb_Filt/1
  ProbCalculat/1(PIL_ObjinEgoLaneProb_Filt) -> PIL_ObjinEgoLaneProb_Filt/1
  Bus Selector8/2 -> BoundaryCalculat/2(TOS_AddAttributes)  "<TOS_PP_AddAttributes_bus>"
  Bus Selector8/1 -> BoundaryCalculat/1(OFM_SignalVerification)  "<OFM_SignalVerification>"
  Bus Selector8/5 -> BoundaryCalculat/5(PP_Right_CenterLine)  "<PP_RightLane_CenterLine>"
  Bus Selector8/4 -> BoundaryCalculat/4(PP_Left_CenterLine)  "<PP_LeftLane_CenterLine>"
  Bus Selector8/3 -> BoundaryCalculat/3(PP_Same_CenterLine)  "<PP_EgoLane_CenterLine>"
  PP_CenterLineCalculat/1 -> Bus Creator1/2
  "OFM_SignalVerification "/1 -> Bus Creator1/4
  VIE_SignalVerification/1 -> Bus Creator1/3
  TOS_AddAttributes/1 -> Bus Creator1/1
  Bus Selector2/1 -> PIL_ObjectToCenterLine_dy_Filt/1(ObjectToCenterLine_dy)  "<PP_ObjectToCenterLine_dy>"
  Bus Selector2/3 -> PIL_ObjectToCenterLine_dy_Filt/3(Object_ID)  "<Object_ID>"
  Bus Selector7/4 -> ProbCalculat/4(LM_SignalVerification)  "<LM_SignalVerification>"
  ProbCalculat/5(PIL_EgoVehicleProFilt) -> PIL_EgoVehicleProFilt/1
  ProbCalculat/4("PIL_ObjLaneProb_all ") -> "PIL_ObjLaneProb_all "/1
  Bus Selector6/5 -> OverlapRatio_Calculate/5(Object_Type)  "<Object_Type>"

== system PubIfDecisionTOS_MDL/TOS_20201112/TOS_2012080320/PP1128 ==
  OFMInfo : Inport
  vxvRefMs : Inport  Port=2  OutDataTypeStr=single
  psiDtOpt : Inport  Port=3  OutDataTypeStr=single  Interpolate=off
  kapTraj : Inport  Port=4  OutDataTypeStr=single
  axvRefMs2 : Inport  Port=5  OutDataTypeStr=single
  TOS_VC AN_CSA : Inport  Port=6  BusOutputAsStruct=on
  LM_LINE_LL : Inport  Port=7  BusOutputAsStruct=on
  LM_LINE_LR : Inport  Port=8  BusOutputAsStruct=on
  LM_LINE_RL : Inport  Port=9  BusOutputAsStruct=on
  LM_LINE_RR : Inport  Port=10  BusOutputAsStruct=on
  LM_SpecialRoadType : Inport  Port=11  OutDataTypeStr=uint8  PortDimensions=1  BusOutputAsStruct=on
  LM_RoadNumChgType : Inport  Port=12  OutDataTypeStr=uint8  PortDimensions=1  BusOutputAsStruct=on
  LM_DrivInWLType : Inport  Port=13  OutDataTypeStr=uint8  PortDimensions=1  BusOutputAsStruct=on
  AAT-AdditionalAttributes : Subsystem
  ISV_InputSignalVerification : Subsystem
  TOS_AddAttributes : Outport
  PP_CenterLineCalculat : Outport  Port=2
  VIE_SignalVerification : Outport  Port=3
  OFM_SignalVerification : Outport  Port=4
  LM_SignalVerification : Outport  Port=5
  TOS_VCAN_SignalVerification : Outport  Port=6
  PP_REElementType : Outport  Port=7
  wires:
  OFMInfo/1 -> ISV_InputSignalVerification/1(OFMInfo)
  psiDtOpt/1 -> ISV_InputSignalVerification/3(psiDtOpt)
  vxvRefMs/1 -> ISV_InputSignalVerification/2(vxvRefMs)  "vxvRefMs"
  ISV_InputSignalVerification/1(LM_SignalVerification) -> LM_SignalVerification/1, AAT-AdditionalAttributes/1(LM_SignalVerification)
  ISV_InputSignalVerification/2(OFM_SignalVerification) -> AAT-AdditionalAttributes/2(OFM_Info)
  ISV_InputSignalVerification/3(VIE_SignalVerification) -> VIE_SignalVerification/1, AAT-AdditionalAttributes/3(VIE_SignalVerification)
  AAT-AdditionalAttributes/1(TOS_AddAttributes) -> TOS_AddAttributes/1
  kapTraj/1 -> ISV_InputSignalVerification/4(kapTraj)
  TOS_VC AN_CSA/1 -> ISV_InputSignalVerification/6(TOS_VCAN_CSA)
  axvRefMs2/1 -> ISV_InputSignalVerification/5(axvRefMs2)  "axvRefMs2"
  LM_LINE_LL/1 -> ISV_InputSignalVerification/7(LM_LINE_LL)
  LM_LINE_LR/1 -> ISV_InputSignalVerification/8(LM_LINE_LR)
  LM_LINE_RL/1 -> ISV_InputSignalVerification/9(LM_LINE_RL)
  LM_LINE_RR/1 -> ISV_InputSignalVerification/10(LM_LINE_RR)
  LM_SpecialRoadType/1 -> ISV_InputSignalVerification/11(LM_SpecialRoadType)
  LM_RoadNumChgType/1 -> ISV_InputSignalVerification/12(LM_RoadNumChgType)
  LM_DrivInWLType/1 -> ISV_InputSignalVerification/13(LM_DrivInWLType)
  AAT-AdditionalAttributes/2(PP_CenterLineCalculat) -> PP_CenterLineCalculat/1
  ISV_InputSignalVerification/4(TOS_VCAN_SignalVerification) -> TOS_VCAN_SignalVerification/1
  AAT-AdditionalAttributes/3(OFM_SignalVerification) -> OFM_SignalVerification/1
  AAT-AdditionalAttributes/4(PP_REElementType) -> PP_REElementType/1
